simulink model "Robot_3gdl_PRR_DinInv"  (R2014a)
settings: Solver=ode3  StartTime=0.0  StopTime=9.99  FixedStep=0.03  RelTol=1e-3
values from neighbouring files (symbols this model uses):
  RobotPRR = SerialLink(L,'name','PRR')    [IniciaParametrosPRR.m]
libraries: roblocks x3
settings Model: Creator=corkep  LastModifiedBy=fertape
settings DataIOCC: SignalLoggingSaveFormat=ModelDataLogs
settings OptimizationCC: ExpressionDepthLimit=2147483647
settings DebuggingCC: UnderspecifiedInitializationDetection=Classic  FcnCallInpInsideContextMsg=UseLocalSettings  StateNameClashWarn=warning
settings GRTTargetCC: CombineOutputUpdateFcns=off  GRTInterface=on

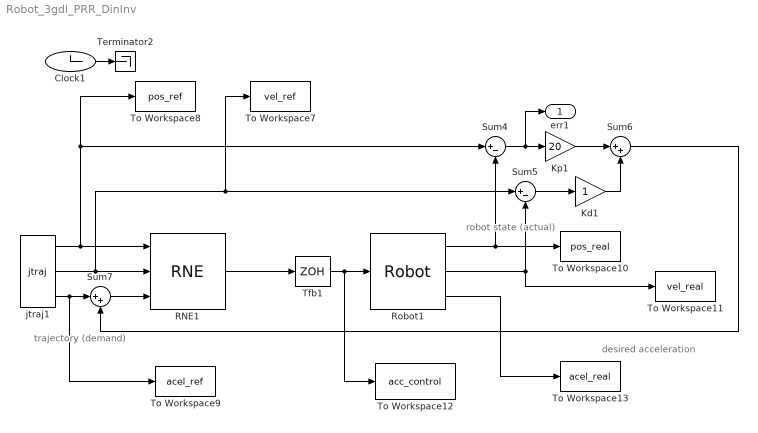
== system Robot_3gdl_PRR_DinInv ==
  note: trajectory
      | (demand)
  note: robot state
      | (actual)
  note: desired acceleration
  Clock1 : Clock
  Kd1 : Gain  SaturateOnIntegerOverflow=on  OutDataTypeStr=Inherit: Same as input  ParamDataTypeStr=Inherit: Same as input
  Kp1 : Gain  Gain=20  SaturateOnIntegerOverflow=on  OutDataTypeStr=Inherit: Same as input  ParamDataTypeStr=Inherit: Same as input
  RNE1 : roblocks/Dynamics/RNE  robot=RobotPRR.nofriction()  grav=gravedad
  Robot1 : roblocks/Dynamics/Robot  robot=RobotPRR  q0=Qini
  Sum4 : Sum  Inputs=|+-  SaturateOnIntegerOverflow=on  InputSameDT=on  OutDataTypeStr=Inherit: Same as first input
  Sum5 : Sum  Inputs=|+-  SaturateOnIntegerOverflow=on  InputSameDT=on  OutDataTypeStr=Inherit: Same as first input
  Sum6 : Sum  Inputs=|++  SaturateOnIntegerOverflow=on  InputSameDT=on  OutDataTypeStr=Inherit: Same as first input
  Sum7 : Sum  Inputs=|++  SaturateOnIntegerOverflow=on  InputSameDT=on  OutDataTypeStr=Inherit: Same as first input
  Terminator2 : Terminator
  Tfb1 : ZeroOrderHold  SampleTime=0.03
  To Workspace10 : ToWorkspace  VariableName=pos_real  SaveFormat=Structure With Time  SampleTime=-1
  To Workspace11 : ToWorkspace  VariableName=vel_real  SaveFormat=Structure With Time  SampleTime=-1
  To Workspace12 : ToWorkspace  VariableName=acc_control  SaveFormat=Structure With Time  SampleTime=-1
  To Workspace13 : ToWorkspace  VariableName=acel_real  SaveFormat=Structure With Time  SampleTime=-1
  To Workspace7 : ToWorkspace  VariableName=vel_ref  SaveFormat=Structure With Time  SampleTime=-1
  To Workspace8 : ToWorkspace  VariableName=pos_ref  SaveFormat=Structure With Time  SampleTime=-1
  To Workspace9 : ToWorkspace  VariableName=acel_ref  SaveFormat=Structure With Time  SampleTime=-1
  jtraj1 : roblocks/Trajectory/jtraj  q0=Qini  qf=Qfin  tmax=10  ts=0.03
  err1 : Outport
  wires:
  Sum4/1 -> Kp1/1, err1/1
  Kp1/1 -> Sum6/1
  Robot1/1 -> Sum4/2, To Workspace10/1
  Robot1/2 -> To Workspace11/1, Sum5/2
  RNE1/1 -> Tfb1/1
  jtraj1/1 -> To Workspace8/1, Sum4/1, RNE1/1
  jtraj1/2 -> To Workspace7/1, Sum5/1, RNE1/2
  Sum5/1 -> Kd1/1
  Kd1/1 -> Sum6/2
  jtraj1/3 -> To Workspace9/1, Sum7/1
  Robot1/3 -> To Workspace13/1
  Clock1/1 -> Terminator2/1
  Sum7/1 -> RNE1/3
  Sum6/1 -> Sum7/2
  Tfb1/1 -> To Workspace12/1, Robot1/1
